simulink model "WIP_nl_model"  (R2025b)
settings: Solver=ode23t  StartTime=0.0  StopTime=10.0  MaxStep=1e-3  RelTol=1e-3
undefined symbols (not defined in the file): g, k1, k2, k3, p0
libraries: simulink_extras x2
settings Model: Creator=upattacini  LastModifiedBy=upattacini
settings DataIOCC: SaveOutput=off  DSMLogging=off  SaveTime=off

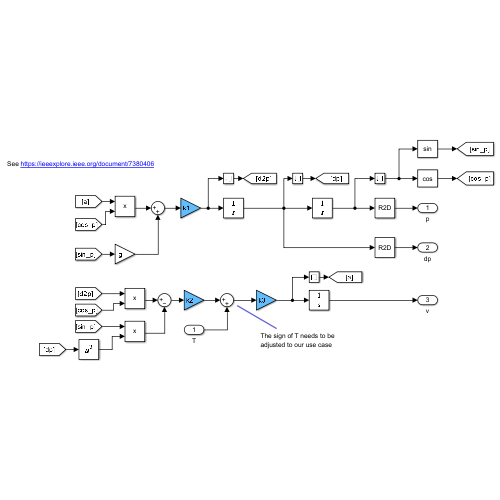
[thumbnail: Simulink's stored preview of the top-level diagram]
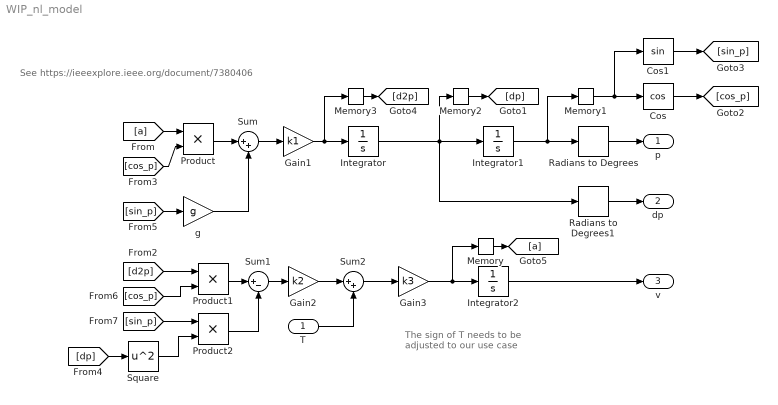
== system WIP_nl_model ==
  note: The sign of T needs to be
      | adjusted to our use case
  note: See https://ieeexplore.ieee.org/document/7380406
  T : Inport
  Cos : Trigonometry  Operator=cos
  Cos1 : Trigonometry
  Gain1 : Gain  Gain=k1
  Gain2 : Gain  Gain=k2
  Gain3 : Gain  Gain=k3
  Integrator : Integrator  ContinuousStateAttributes='dp'
  Integrator1 : Integrator  InitialCondition=p0 * pi/180  ContinuousStateAttributes='p'
  Integrator2 : Integrator  ContinuousStateAttributes='v'
  Memory : Memory  InheritSampleTime=on  LinearizeMemory=on  LinearizeAsDelay=on
  Memory1 : Memory  InitialCondition=p0 * pi/180  InheritSampleTime=on  LinearizeMemory=on  LinearizeAsDelay=on
  Memory2 : Memory  InheritSampleTime=on  LinearizeMemory=on  LinearizeAsDelay=on
  Memory3 : Memory  InheritSampleTime=on  LinearizeMemory=on  LinearizeAsDelay=on
  Product : Product
  Product1 : Product
  Product2 : Product
  Radians to Degrees : simulink_extras/Transformations/Radians to Degrees
  Radians to Degrees1 : simulink_extras/Transformations/Radians to Degrees
  Square : Math  Operator=square
  Sum : Sum  Inputs=|++
  Sum1 : Sum  Inputs=|+-
  Sum2 : Sum  Inputs=|++
  g : Gain  Gain=g
  p : Outport
  dp : Outport  Port=2
  v : Outport  Port=3
  wires:
  Radians to Degrees/1 -> p/1
  Integrator/1 -> Radians to Degrees1/1, Memory2/1, Integrator1/1
  Cos1/1 -> [sin_p]
  Gain3/1 -> Integrator2/1, Memory/1
  [sin_p] -> Product2/1
  Radians to Degrees1/1 -> dp/1
  Product1/1 -> Sum1/1
  Memory/1 -> [a]
  [cos_p] -> Product/2
  T/1 -> Sum2/2
  Sum2/1 -> Gain3/1
  Integrator1/1 -> Radians to Degrees/1, Memory1/1
  Memory3/1 -> [d2p]
  Product/1 -> Sum/1
  Memory2/1 -> [dp]
  [sin_p] -> g/1
  [a] -> Product/1
  Gain1/1 -> Memory3/1, Integrator/1
  Gain2/1 -> Sum2/1
  Product2/1 -> Sum1/2
  Sum/1 -> Gain1/1
  Cos/1 -> [cos_p]
  Sum1/1 -> Gain2/1
  [cos_p] -> Product1/2
  g/1 -> Sum/2
  Square/1 -> Product2/2
  Integrator2/1 -> v/1
  [dp] -> Square/1
  [d2p] -> Product1/1
  Memory1/1 -> Cos1/1, Cos/1
